simulink model "Dyn_6DoF_v2_0_R2015B"  (R2015b)
settings: Solver=ode4  SolverMode=SingleTasking  StartTime=0.0  StopTime=simInit.TSIM  FixedStep=simInit.dt  MaxStep=simInit.dt  RelTol=1e-3
InitFcn:
  | close all
undefined symbols (not defined in the file): act, base_windspeed, constr, DE2019, DiscIntNeverNeededParam, ENVMT, Lbooth, loiterStates, omega_rate_max, params, simInit, T, winchParameter
libraries: simulink x41, simulink_extras x4, dspsigops x1
(part 3 of 6)

== system Dyn_6DoF_v2_0_R2015B/AirborneSystem/FlightControlSystem/AttitudeAndRateLoop/AttitudeController/SecondOrderReferenceModel_alpha_a ==
  y_cmd : Inport
  hedge : Inport  Port=2
  Constant5 : Constant  Value=omega0_max
  Discrete-Time Integrator : DiscreteIntegrator  InitialConditionSetting=State (most efficient)  SampleTime=-1  LimitOutput=on  UpperSaturationLimit=y_max  LowerSaturationLimit=y_min  ICPrevOutput=DiscIntNeverNeededParam  ICPrevScaledInput=DiscIntNeverNeededParam
  Discrete-Time Integrator1 : DiscreteIntegrator  InitialConditionSetting=State (most efficient)  SampleTime=-1  LimitOutput=on  UpperSaturationLimit=yd_max  LowerSaturationLimit=yd_min  ICPrevOutput=DiscIntNeverNeededParam  ICPrevScaledInput=DiscIntNeverNeededParam
  Gain2 : Gain  Gain=2*zeta0
  Product : Product  Inputs=3
  Product1 : Product
  Saturation : Saturate  UpperLimit=y_max  LowerLimit=y_min
  Saturation1 : Saturate  UpperLimit=y2d_max  LowerLimit=y2d_min
  Sum : Sum  Inputs=|+-
  Sum1 : Sum  Inputs=|+-
  Sum2 : Sum  Inputs=|+-
  y_ref : Outport
  y_ref_dot : Outport  Port=2
  wires:
  Product/1 -> Sum/1
  Sum/1 -> Saturation1/1
  y_cmd/1 -> Saturation/1
  Saturation1/1 -> Discrete-Time Integrator1/1
  Gain2/1 -> Sum/2
  Sum1/1 -> Product/2
  Discrete-Time Integrator/1 -> Sum1/2, y_ref/1
  Discrete-Time Integrator1/1 -> y_ref_dot/1, Product1/1, Sum2/1
  Saturation/1 -> Sum1/1
  Sum2/1 -> Discrete-Time Integrator/1
  hedge/1 -> Sum2/2
  Product1/1 -> Gain2/1
  Constant5/1 -> Product1/2, Product/3, Product/1

== system Dyn_6DoF_v2_0_R2015B/AirborneSystem/FlightControlSystem/AttitudeAndRateLoop/AttitudeController/SecondOrderReferenceModel_mu_a ==
  y_cmd : Inport
  hedge : Inport  Port=2
  Constant5 : Constant  Value=omega0_max
  Discrete-Time Integrator : DiscreteIntegrator  InitialConditionSetting=State (most efficient)  SampleTime=-1  LimitOutput=on  UpperSaturationLimit=y_max  LowerSaturationLimit=y_min  ICPrevOutput=DiscIntNeverNeededParam  ICPrevScaledInput=DiscIntNeverNeededParam
  Discrete-Time Integrator1 : DiscreteIntegrator  InitialConditionSetting=State (most efficient)  SampleTime=-1  LimitOutput=on  UpperSaturationLimit=yd_max  LowerSaturationLimit=yd_min  ICPrevOutput=DiscIntNeverNeededParam  ICPrevScaledInput=DiscIntNeverNeededParam
  Gain2 : Gain  Gain=2*zeta0
  Product : Product  Inputs=3
  Product1 : Product
  Saturation : Saturate  UpperLimit=y_max  LowerLimit=y_min
  Saturation1 : Saturate  UpperLimit=y2d_max  LowerLimit=y2d_min
  Sum : Sum  Inputs=|+-
  Sum1 : Sum  Inputs=|+-
  Sum2 : Sum  Inputs=|+-
  y_ref : Outport
  y_ref_dot : Outport  Port=2
  wires:
  Discrete-Time Integrator/1 -> Sum1/2, y_ref/1
  Product/1 -> Sum/1
  y_cmd/1 -> Saturation/1
  Discrete-Time Integrator1/1 -> y_ref_dot/1, Product1/1, Sum2/1
  Sum/1 -> Saturation1/1
  Gain2/1 -> Sum/2
  Sum1/1 -> Product/2
  Saturation1/1 -> Discrete-Time Integrator1/1
  Saturation/1 -> Sum1/1
  Sum2/1 -> Discrete-Time Integrator/1
  hedge/1 -> Sum2/2
  Product1/1 -> Gain2/1
  Constant5/1 -> Product1/2, Product/3, Product/1

== system Dyn_6DoF_v2_0_R2015B/AirborneSystem/FlightControlSystem/AttitudeAndRateLoop/RateLoop/Actuatormodel _SS_2 ==
  u_cmd : Inport
  Aileron1 : Subsystem  mask(Rate and Position Limited Servo){freq=act.aileron.w0/(2*pi), RL=act.aileron.rl, POS_hi=act.aileron.max_deflection, POS_lo=act.aileron.min_deflection, Bias=act.aileron.bias}
      mask prompts: freq "Bandwidth, Hz"; RL "Rate Limit:"; POS_hi "Position Limit High:"; POS_lo "Position Limit Low:"; Bias "Bias Value:"
      mask help:
      | First order transfer function: w/(s+w), with rate and position limits
      | and output bias level.
      mask Display:
      | text(.48,.55,sprintf('%3.1f Hz\nBW',freq),'horizontalAlignment','center');
      | 
      | text(0.18,0.45,sprintf('|d/dt|\n<%0.1f',RL),'horizontalAlignment','center');
      | 
      | text(0.88,0.85,num2str(POS_hi),'horizontalAlignment', 'center');
      | text(0.88,0.2,num2str(POS_lo),'horizontalAlignment', 'center');
      | text(0.73,0.5,'P\nL');
      | 
      | 
      | plot([0.83 0.87 0.93 0.97],[0.4 0.4 0.6 0.6]);
      | plot([0.81 0.99],[0.5 0.5]);
      | plot([0.9 0.9],[0.3 0.7]);
      | plot([0.81 0.99 0.99 0.81 0.81],[0.3 0.3 0.7 0.7 0.3]);
  Delay1 : Delay  Commented=on  DelayLength=1  InitialCondition=0
  Delay2 : Delay  Commented=on  DelayLength=1  InitialCondition=0
  Delay3 : Delay  Commented=on  DelayLength=1  InitialCondition=0
  Delay4 : Delay  DelayLength=1  InitialCondition=0
  Delay5 : Delay  DelayLength=1  InitialCondition=0
  Delay6 : Delay  DelayLength=1  InitialCondition=0
  Demux : Demux  Outputs=3
  Elevator : Subsystem  mask(Rate and Position Limited Servo){freq=act.elevator.w0/(2*pi), RL=act.elevator.rl, POS_hi=act.elevator.max_deflection, POS_lo=act.elevator.min_deflection, Bias=act.elevator.bias}
      mask prompts: freq "Bandwidth, Hz"; RL "Rate Limit:"; POS_hi "Position Limit High:"; POS_lo "Position Limit Low:"; Bias "Bias Value:"
      mask help:
      | First order transfer function: w/(s+w), with rate and position limits
      | and output bias level.
      mask Display:
      | text(.48,.55,sprintf('%3.1f Hz\nBW',freq),'horizontalAlignment','center');
      | 
      | text(0.18,0.45,sprintf('|d/dt|\n<%0.1f',RL),'horizontalAlignment','center');
      | 
      | text(0.88,0.85,num2str(POS_hi),'horizontalAlignment', 'center');
      | text(0.88,0.2,num2str(POS_lo),'horizontalAlignment', 'center');
      | text(0.73,0.5,'P\nL');
      | 
      | 
      | plot([0.83 0.87 0.93 0.97],[0.4 0.4 0.6 0.6]);
      | plot([0.81 0.99],[0.5 0.5]);
      | plot([0.9 0.9],[0.3 0.7]);
      | plot([0.81 0.99 0.99 0.81 0.81],[0.3 0.3 0.7 0.7 0.3]);
  Manual Switch : ManualSwitch  CurrentSetting=0
  Mux1 : Mux  Inputs=3
  Mux2 : Mux  Inputs=3
  Rudder1 : Subsystem  mask(Rate and Position Limited Servo){freq=act.rudder.w0/(2*pi), RL=act.rudder.rl, POS_hi=act.rudder.max_deflection, POS_lo=act.rudder.min_deflection, Bias=act.rudder.bias}
      mask prompts: freq "Bandwidth, Hz"; RL "Rate Limit:"; POS_hi "Position Limit High:"; POS_lo "Position Limit Low:"; Bias "Bias Value:"
      mask help:
      | First order transfer function: w/(s+w), with rate and position limits
      | and output bias level.
      mask Display:
      | text(.48,.55,sprintf('%3.1f Hz\nBW',freq),'horizontalAlignment','center');
      | 
      | text(0.18,0.45,sprintf('|d/dt|\n<%0.1f',RL),'horizontalAlignment','center');
      | 
      | text(0.88,0.85,num2str(POS_hi),'horizontalAlignment', 'center');
      | text(0.88,0.2,num2str(POS_lo),'horizontalAlignment', 'center');
      | text(0.73,0.5,'P\nL');
      | 
      | 
      | plot([0.83 0.87 0.93 0.97],[0.4 0.4 0.6 0.6]);
      | plot([0.81 0.99],[0.5 0.5]);
      | plot([0.9 0.9],[0.3 0.7]);
      | plot([0.81 0.99 0.99 0.81 0.81],[0.3 0.3 0.7 0.7 0.3]);
  Saturation : Saturate  Commented=on  UpperLimit=act.aileron.max_deflection  LowerLimit=act.aileron.min_deflection
  Saturation1 : Saturate  Commented=on  UpperLimit=act.elevator.max_deflection  LowerLimit=act.elevator.min_deflection
  Saturation2 : Saturate  Commented=on  UpperLimit=act.rudder.max_deflection  LowerLimit=act.rudder.min_deflection
  Saturation4 : Saturate  UpperLimit=act.elevator.max_deflection  LowerLimit=act.elevator.min_deflection
  Saturation6 : Saturate  UpperLimit=act.aileron.max_deflection  LowerLimit=act.aileron.min_deflection
  Saturation7 : Saturate  UpperLimit=act.rudder.max_deflection  LowerLimit=act.rudder.min_deflection
  Act_out_est : Outport
  wires:
  Delay3/1 -> Saturation2/1
  Mux2/1 -> Manual Switch/2
  Saturation1/1 -> Mux1/2
  Delay4/1 -> Saturation6/1
  Delay1/1 -> Saturation/1
  Manual Switch/1 -> Act_out_est/1
  Saturation6/1 -> Aileron1/1(In)
  Saturation/1 -> Mux1/1
  Saturation7/1 -> Rudder1/1(In)
  Rudder1/1(Out) -> Mux2/3
  Elevator/1(Out) -> Mux2/2
  Delay5/1 -> Saturation4/1
  Demux/2 -> Delay5/1, Delay2/1
  Mux1/1 -> Manual Switch/1
  Demux/1 -> Delay1/1, Delay4/1
  Delay6/1 -> Saturation7/1
  Delay2/1 -> Saturation1/1
  Saturation4/1 -> Elevator/1(In)
  Saturation2/1 -> Mux1/3
  u_cmd/1 -> Demux/1
  Aileron1/1(Out) -> Mux2/1
  Demux/3 -> Delay6/1, Delay3/1

== system Dyn_6DoF_v2_0_R2015B/AirborneSystem/FlightControlSystem/AttitudeAndRateLoop/RateLoop/ControlAllocation ==
  deflections_actuator_output : Inport
  airdata : Inport  Port=2
  Delta_mom_cmd : Inport  Port=3
  Constant1 : Constant  Value=1e-6
  Gain14 : Gain  Gain=[1/ DE2019.b, 0, 0; 0, 1/ DE2019.c, 0; 0, 0, 1/ DE2019.b]  Multiplication=Matrix(K*u)
  Gain15 : Gain  Gain=DE2019.S_wing
  Gain3 : Gain  Gain=0.5*ENVMT.rhos
  Product : Product  Inputs=*/
  Product2 : Product
  Selector : Selector  InputPortWidth=3  IndexOptions=Index vector (dialog)  Indices=1  OutputSizes=1
  Selector1 : Selector  InputPortWidth=3  IndexOptions=Index vector (dialog)  Indices=2  OutputSizes=1
  Sum13 : Sum
  Sum2 : Sum  Inputs=|++
  allocation : MATLAB Function  TreatAsAtomicUnit=on
  deflections_cmd : Outport
  wires:
  Selector1/1 -> allocation/2(alpha)
  airdata/1 -> Selector/1, Selector1/1
  Product2/1 -> Gain3/1
  Selector/1 -> Product2/1, Product2/2
  deflections_actuator_output/1 -> Sum13/1
  Gain14/1 -> allocation/1(dC_pqr)
  Sum13/1 -> deflections_cmd/1
  allocation/1(Delta_deltas) -> Sum13/2
  Sum2/1 -> Product/2
  Constant1/1 -> Sum2/2
  Gain3/1 -> Gain15/1
  Gain15/1 -> Sum2/1
  Product/1 -> Gain14/1
  Delta_mom_cmd/1 -> Product/1

== system Dyn_6DoF_v2_0_R2015B/AirborneSystem/FlightControlSystem/AttitudeAndRateLoop/RateLoop/Rate_Loop ==
  omega_OB_B : Inport
  omega_OB_B_cmd : Inport  Port=2  PortDimensions=[3,1]
  M_a_B_est : Inport  Port=3  PortDimensions=[3,1]
  Demux1 : Demux  Commented=on  Outputs=3
  Demux2 : Demux  Commented=on  Outputs=3
  Demux3 : Demux  Commented=on  Outputs=3
  Gain : Gain  Commented=on  Gain=180/pi
  Gain1 : Gain  Commented=on  Gain=180/pi
  Gain2 : Gain  Commented=on  Gain=180/pi
  Hedging : Subsystem
  InversionRotationalDynamics : MATLAB Function  TreatAsAtomicUnit=on
  Mux{,1..2,4} (4 alike) : Mux  Commented=on  Inputs=3
  NonlinearDynamicInversion : Subsystem
  Scope : Scope  Commented=on  NumInputPorts=3
  Selector : Selector  InputPortWidth=3  IndexOptions=Index vector (dialog)  Indices=1  OutputSizes=1
  Selector1 : Selector  InputPortWidth=3  IndexOptions=Index vector (dialog)  Indices=2  OutputSizes=1
  Selector2 : Selector  InputPortWidth=3  IndexOptions=Index vector (dialog)  Indices=3  OutputSizes=1
  Sum1 : Sum  Inputs=|+-
  Sum12 : Sum  Inputs=-+
  Sum2 : Sum  Inputs=|+-
  Sum3 : Sum  Inputs=|+-
  To Workspace11 : ToWorkspace  Commented=on  VariableName=omega_OB_B_cmds  SaveFormat=Timeseries  SampleTime=-1
  delta_M_cmd : Outport
  wires:
  Mux2/1 -> To Workspace11/1
  omega_OB_B_cmd/1 -> Demux2/1, NonlinearDynamicInversion/5(omega_OB_B_cmd)
  Selector/1 -> Sum2/1
  Selector1/1 -> Sum1/1
  Selector2/1 -> Sum3/1
  NonlinearDynamicInversion/1(omega_OB_ref) -> Demux1/1
  Sum3/1 -> NonlinearDynamicInversion/1(r_h)
  Sum1/1 -> NonlinearDynamicInversion/2(q_h)
  Sum2/1 -> NonlinearDynamicInversion/3(p_h)
  Hedging/3(nu_r_hat) -> Sum3/2
  Hedging/2(nu_q_hat) -> Sum1/2
  Hedging/1(nu_p_hat) -> Sum2/2
  Sum12/1 -> delta_M_cmd/1
  InversionRotationalDynamics/1(M_des) -> Sum12/2
  M_a_B_est/1 -> Hedging/1(Torque_estimate), Sum12/1
  Gain1/1 -> Scope/2
  Mux/1 -> Gain/1, Mux2/1
  Mux1/1 -> Gain1/1, Mux2/2
  Demux1/1 -> Mux/2
  Demux1/2 -> Mux1/2
  Demux1/3 -> Mux4/2
  Mux4/1 -> Gain2/1, Mux2/3
  Gain2/1 -> Scope/3
  Gain/1 -> Scope/1
  Demux2/1 -> Mux/1
  Demux2/2 -> Mux1/1
  Demux2/3 -> Mux4/1
  Demux3/1 -> Mux/3
  Demux3/2 -> Mux1/3
  Demux3/3 -> Mux4/3
  omega_OB_B/1 -> Demux3/1, Hedging/2(rates), InversionRotationalDynamics/1(omega_OB_B), NonlinearDynamicInversion/4(omega_OB_B)
  NonlinearDynamicInversion/2(nu_NDI) -> Selector/1, Selector1/1, Selector2/1, InversionRotationalDynamics/2(nu_NDI)

== system Dyn_6DoF_v2_0_R2015B/AirborneSystem/FlightControlSystem/PathFollowingController_SS_3/FlightOnFlatEarth (Retraction&Loitering)/CalculateAttitudeCmds ==
  flight_on_flatearth_flag : Inport
  pathangles_k_cmd : Inport  Port=2
  Ft_set : Inport  Port=3
  F_t_kite : Inport  Port=4
  sub_flightMode : Inport  Port=5
  flightMode : Inport  Port=6
  StateEstimation_Bus : Inport  Port=7
  Demux : Demux  Outputs=3
  FlightPathLoopRetraction_Aerodynamic : Subsystem
  Mux1 : Mux  Inputs=3
  Signal Specification : SignalSpecification  Dimensions=[3,1]
  Terminator2 : Terminator
  mu_a_cmd : Outport
  alpha_cmd : Outport  Port=2
  wires:
  StateEstimation_Bus/1 -> FlightPathLoopRetraction_Aerodynamic/4(StateEstimation_Bus)
  Demux/3 -> Terminator2/1
  Demux/2 -> alpha_cmd/1
  flight_on_flatearth_flag/1 -> FlightPathLoopRetraction_Aerodynamic/Enable
  FlightPathLoopRetraction_Aerodynamic/2(alpha_a_cmd) -> Mux1/2
  flightMode/1 -> FlightPathLoopRetraction_Aerodynamic/1(flight_mode)
  Signal Specification/1 -> Demux/1
  Demux/1 -> mu_a_cmd/1
  Mux1/1 -> Signal Specification/1
  F_t_kite/1 -> FlightPathLoopRetraction_Aerodynamic/3(F_t_kite)
  FlightPathLoopRetraction_Aerodynamic/1(mu_a_cmd) -> Mux1/1
  Ft_set/1 -> FlightPathLoopRetraction_Aerodynamic/2(F_t_set)
  FlightPathLoopRetraction_Aerodynamic/3(beta_a_cmd) -> Mux1/3
  pathangles_k_cmd/1 -> FlightPathLoopRetraction_Aerodynamic/5(kinematic_path_cmd)
  sub_flightMode/1 -> FlightPathLoopRetraction_Aerodynamic/6(sub_flightMode)

== system Dyn_6DoF_v2_0_R2015B/AirborneSystem/FlightControlSystem/PathFollowingController_SS_3/FlightOnFlatEarth (Retraction&Loitering)/GuidanceFlatEarth ==
  flightMode : Inport
  StateEstimation_Bus : Inport  Port=2
  reset_flat : Inport  Port=3
  V_ro : Inport  Port=4
  Tether_length : Inport  Port=5
  Enable : EnablePort
  Bus Selector : BusSelector  OutputSignals=pos_G_O_m,vel_K_O_mDs,pathangles_k,pos_G_W
  Compare To Constant : simulink/Logic and Bit Operations/Compare To Constant  relop===  const=6  OutDataTypeStr=boolean
  Compare To Constant2 : simulink/Logic and Bit Operations/Compare To Constant  relop===  const=6  OutDataTypeStr=boolean
  LoiteringGuidance : Subsystem
  Retraction_Nav : Subsystem
  Switch1 : Switch  Criteria=u2 > Threshold
  distances2slope : Outport
  course_path : Outport  Port=2
  valid_transition_region : Outport  Port=3
  transition_flag : Outport  Port=4
  flag_pos_W : Outport  Port=5
  transition_x_target : Outport  Port=6
  Vk_desired_retraction : Outport  Port=7
  arcP : Outport  Port=8
  wires:
  Bus Selector/1 -> Retraction_Nav/1(pos_O), LoiteringGuidance/2(pos_G_O_m)  "<pos_G_O_m>"
  StateEstimation_Bus/1 -> Bus Selector/1
  Bus Selector/2 -> Retraction_Nav/2(vel_k_O), LoiteringGuidance/3(vel_K_O_mDs)  "<vel_K_O_mDs>"
  Compare To Constant2/1 -> Retraction_Nav/Enable
  Switch1/1 -> course_path/1
  Compare To Constant/1 -> Switch1/2
  Retraction_Nav/1(distances2slope) -> distances2slope/1
  Retraction_Nav/7(path_k_cmds) -> Switch1/1
  flightMode/1 -> LoiteringGuidance/1(flightMode), Compare To Constant/1, Compare To Constant2/1
  Bus Selector/3 -> LoiteringGuidance/4(pathangles_k)  "<pathangles_k>"
  LoiteringGuidance/1(path_k_cmds) -> Switch1/3
  LoiteringGuidance/2(valid_transition_region) -> valid_transition_region/1
  Retraction_Nav/2(transition_flag) -> transition_flag/1
  reset_flat/1 -> LoiteringGuidance/6(reset_flag)
  Bus Selector/4 -> LoiteringGuidance/5(pos_W)  "<pos_G_W>"
  Retraction_Nav/3(flag_pos_y_W) -> flag_pos_W/1
  Retraction_Nav/4(transition_x_target) -> transition_x_target/1
  Retraction_Nav/5(Vk_desired_retraction) -> Vk_desired_retraction/1
  V_ro/1 -> Retraction_Nav/3(V_ro)
  Tether_length/1 -> Retraction_Nav/4(Tether_length)
  Retraction_Nav/6(arcP) -> arcP/1

== system Dyn_6DoF_v2_0_R2015B/AirborneSystem/FlightControlSystem/PathFollowingController_SS_3/FlightOnSphere (Traction)/FlightPathLoopTraction ==
  Ft_set : Inport
  F_a_B_est : Inport  Port=2  PortDimensions=[3,1]
  StateEstimation_Bus : Inport  Port=3
  nu_chi : Inport  Port=4
  nu_gamma : Inport  Port=5
  Enable : EnablePort  StatesWhenEnabling=reset
  Bus Selector : BusSelector  OutputSignals=pos_G_O_m,pathangles_k,v_k_B,airdata,mu_a
  Delay : Delay  DelayLength=1  InitialConditionSource=Input port
      settings: InputPortMap=u0,p4
  Delay1 : Delay  DelayLength=1  InitialConditionSource=Input port
      settings: InputPortMap=u0,p4
  Delay{2..5} (4 alike) : Delay  DelayLength=1
  Demux : Demux  Outputs=2
  Demux1 : Demux  Outputs=2
  Demux2 : Demux  Outputs=2
  EstimatePlantResponse : Subsystem
  MATLAB Function : MATLAB Function  TreatAsAtomicUnit=on
  Mux : Mux  Inputs=2
  Saturation : Saturate  UpperLimit=constr.alpha_a_max  LowerLimit=constr.alpha_a_min
  Sum{,1..3} (4 alike) : Sum  Inputs=|+-
  inversionPathDynamics : MATLAB Function  TreatAsAtomicUnit=on
  mu_a_c_traction : Outport  PortDimensions=1
  alpha_rq : Outport  Port=2  PortDimensions=1
  wires:
  Bus Selector/5 -> Delay/2  "<mu_a>"
  F_a_B_est/1 -> inversionPathDynamics/4(F_a_B_est)
  Demux1/1 -> inversionPathDynamics/6(chi_k)
  inversionPathDynamics/1(mu_a) -> Delay/1, mu_a_c_traction/1
  Mux/1 -> Demux/1
  Demux/2 -> inversionPathDynamics/3(nu_gamma_k)
  Demux/1 -> inversionPathDynamics/2(nu_chi_k)
  inversionPathDynamics/2(mu_k_c) -> EstimatePlantResponse/3(mu_k_sat)
  inversionPathDynamics/3(alpha_rq) -> Saturation/1
  Saturation/1 -> alpha_rq/1, EstimatePlantResponse/2(alpha_rq)
  inversionPathDynamics/4(dphi) -> EstimatePlantResponse/1(dphi)
  Delay1/1 -> inversionPathDynamics/10(L_rq_old)
  Delay/1 -> inversionPathDynamics/11(mu_a_old)
  MATLAB Function/1(L_rq) -> Delay1/2
  inversionPathDynamics/5(L_rq) -> Delay1/1
  Demux1/2 -> inversionPathDynamics/7(gamma_k)
  StateEstimation_Bus/1 -> EstimatePlantResponse/5(StateEstimation_Bus), Bus Selector/1
  Bus Selector/4 -> inversionPathDynamics/9(airdata), MATLAB Function/1(airdata)  "<airdata>"
  Bus Selector/2 -> Demux1/1  "<pathangles_k>"
  Bus Selector/3 -> inversionPathDynamics/8(v_k_B)  "<v_k_B>"
  Bus Selector/1 -> inversionPathDynamics/5(pos_O)  "<pos_G_O_m>"
  Delay5/1 -> Sum3/1
  nu_chi/1 -> Sum/1
  Sum3/1 -> Sum/2
  Delay4/1 -> Sum2/2
  Delay3/1 -> Sum3/2
  Demux2/2 -> Delay4/1
  Sum1/1 -> Mux/2, Delay2/1
  Sum/1 -> Mux/1, Delay5/1
  Delay2/1 -> Sum2/1
  EstimatePlantResponse/1(pathAngleRate) -> Demux2/1
  nu_gamma/1 -> Sum1/1
  Demux2/1 -> Delay3/1
  Sum2/1 -> Sum1/2
  Ft_set/1 -> EstimatePlantResponse/4(Ft), inversionPathDynamics/1(Ft_set)

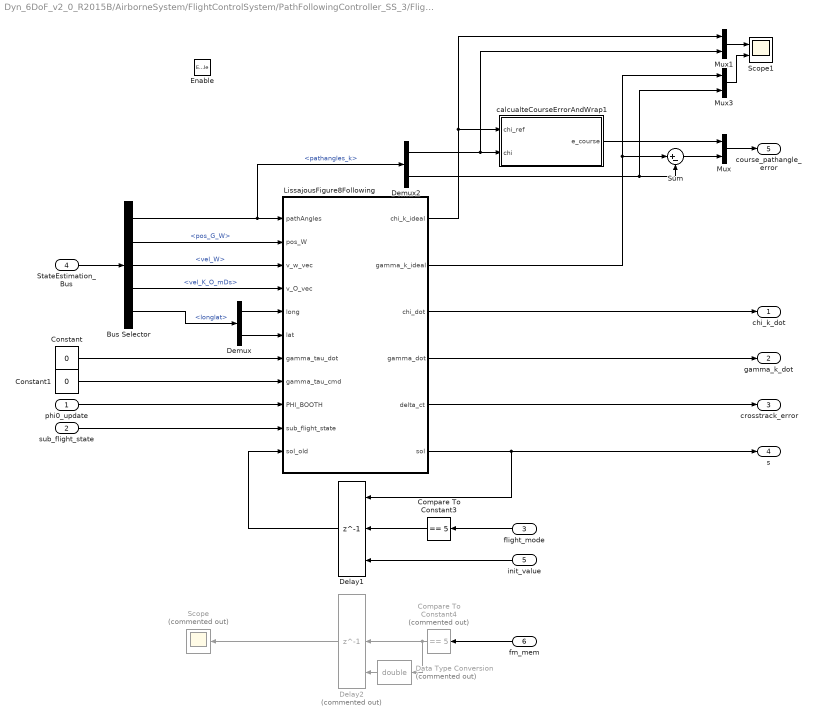
== system Dyn_6DoF_v2_0_R2015B/AirborneSystem/FlightControlSystem/PathFollowingController_SS_3/FlightOnSphere (Traction)/Navigator ==
  phi0_update : Inport
  sub_flight_state : Inport  Port=2
  flight_mode : Inport  Port=3
  StateEstimation_Bus : Inport  Port=4
  init_value : Inport  Port=5
  fm_mem : Inport  Port=6
  Enable : EnablePort  StatesWhenEnabling=reset
  Bus Selector : BusSelector  OutputSignals=pathangles_k,pos_G_W,vel_W,vel_K_O_mDs,longlat
  Compare To Constant3 : simulink/Logic and Bit Operations/Compare To Constant  relop===  const=5  OutDataTypeStr=boolean
  Compare To Constant4 : simulink/Logic and Bit Operations/Compare To Constant  Commented=on  relop===  const=5  OutDataTypeStr=boolean
  Constant : Constant  Value=0
  Constant1 : Constant  Value=0
  Data Type Conversion : DataTypeConversion  Commented=on  OutDataTypeStr=double
  Delay1 : Delay  DelayLength=1  InitialConditionSource=Input port  InitialCondition=pi/2  ExternalReset=Rising
      settings: InputPortMap=u0,r5,p4
  Delay2 : Delay  Commented=on  DelayLength=1  InitialConditionSource=Input port  InitialCondition=pi/2  ExternalReset=Rising
      settings: InputPortMap=u0,r5,p4
  Demux : Demux  Outputs=2
  Demux2 : Demux  Outputs=2
  LissajousFigure8Following : MATLAB Function  TreatAsAtomicUnit=on
  Mux : Mux  Inputs=2
  Mux1 : Mux  Inputs=2
  Mux3 : Mux  Inputs=2
  Scope : Scope  Commented=on
  Scope1 : Scope  NumInputPorts=2
  Sum : Sum  Inputs=|+-
  calcualteCourseErrorAndWrap1 : MATLAB Function  TreatAsAtomicUnit=on
  chi_k_dot : Outport  PortDimensions=1
  gamma_k_dot : Outport  Port=2  PortDimensions=1
  crosstrack_error : Outport  Port=3
  s : Outport  Port=4  PortDimensions=1  InitialOutput=0
  course_pathangle_error : Outport  Port=5
  wires:
  Mux3/1 -> Scope1/2
  Mux1/1 -> Scope1/1
  Delay1/1 -> LissajousFigure8Following/11(sol_old)
  LissajousFigure8Following/6(sol) -> s/1, Delay1/1
  Bus Selector/4 -> LissajousFigure8Following/4(v_O_vec)  "<vel_K_O_mDs>"
  Demux/1 -> LissajousFigure8Following/5(long)
  calcualteCourseErrorAndWrap1/1(e_course) -> Mux/1
  LissajousFigure8Following/1(chi_k_ideal) -> calcualteCourseErrorAndWrap1/1(chi_ref), Mux1/1
  LissajousFigure8Following/2(gamma_k_ideal) -> Sum/1, Mux3/1
  Demux2/1 -> Mux1/2, calcualteCourseErrorAndWrap1/2(chi)
  Demux2/2 -> Mux3/2, Sum/2
  Mux/1 -> course_pathangle_error/1
  LissajousFigure8Following/4(gamma_dot) -> gamma_k_dot/1
  LissajousFigure8Following/3(chi_dot) -> chi_k_dot/1
  Sum/1 -> Mux/2
  Demux/2 -> LissajousFigure8Following/6(lat)
  LissajousFigure8Following/5(delta_ct) -> crosstrack_error/1
  StateEstimation_Bus/1 -> Bus Selector/1
  Bus Selector/2 -> LissajousFigure8Following/2(pos_W)  "<pos_G_W>"
  Bus Selector/5 -> Demux/1  "<longlat>"
  Bus Selector/1 -> Demux2/1, LissajousFigure8Following/1(pathAngles)  "<pathangles_k>"
  flight_mode/1 -> Compare To Constant3/1
  phi0_update/1 -> LissajousFigure8Following/9(PHI_BOOTH)
  Compare To Constant3/1 -> Delay1/2
  init_value/1 -> Delay1/3
  Constant/1 -> LissajousFigure8Following/7(gamma_tau_dot)
  Bus Selector/3 -> LissajousFigure8Following/3(v_w_vec)  "<vel_W>"
  Constant1/1 -> LissajousFigure8Following/8(gamma_tau_cmd)
  Delay2/1 -> Scope/1
  Compare To Constant4/1 -> Delay2/2, Data Type Conversion/1
  fm_mem/1 -> Compare To Constant4/1
  Data Type Conversion/1 -> Delay2/3
  sub_flight_state/1 -> LissajousFigure8Following/10(sub_flight_state)

== system Dyn_6DoF_v2_0_R2015B/AirborneSystem/FlightControlSystem/PathFollowingController_SS_3/FlightOnSphere (Traction)/Pcontroller_ChiGamma_Traction ==
  course_pathangle_error : Inport
  Demux : Demux  Outputs=2
  Kp : Gain  Gain=params.Kp_gamma_k_traction  Multiplication=Matrix(K*u)
  Kp1 : Gain  Gain=params.Kp_chi_k_traction  Multiplication=Matrix(K*u)
  Chi_cntr : Outport
  Gamma_cntr : Outport  Port=2
  wires:
  Kp1/1 -> Chi_cntr/1
  Kp/1 -> Gamma_cntr/1
  course_pathangle_error/1 -> Demux/1
  Demux/2 -> Kp/1
  Demux/1 -> Kp1/1

== system Dyn_6DoF_v2_0_R2015B/AirborneSystem/ForcesAndTorques/aerodynamic forces FSI/Wing Aero/If Action Subsystem ==
  FSI_in : Inport
  simTime : Inport  Port=2
  Action Port : ActionPort
  Demux1 : Demux  Outputs=6
  FSI_sim : MATLABFcn  Commented=on  MATLABFcn=Init_FSIsim  OutputDimensions=[6,1]  Output1D=off
  MATLAB Function : MATLAB Function  TreatAsAtomicUnit=on
  Mux6 : Mux  Inputs=2
  Terminator{1..5,7} (6 alike) : Terminator  Commented=on
  FSI_out : Outport
  wires:
  Demux1/1 -> Terminator7/1  "Fx"
  Demux1/6 -> Terminator1/1  "Myaw"
  simTime/1 -> Mux6/2
  Mux6/1 -> MATLAB Function/1(u)
  Demux1/5 -> Terminator2/1  "Mpitch"
  Demux1/2 -> Terminator3/1  "Fy"
  FSI_in/1 -> Mux6/1
  MATLAB Function/1(y) -> FSI_out/1, Demux1/1
  Demux1/3 -> Terminator5/1  "Fz"
  Demux1/4 -> Terminator4/1  "Mroll"

== system Dyn_6DoF_v2_0_R2015B/AirborneSystem/ForcesAndTorques/aerodynamic forces FSI/Wing Aero/If Action Subsystem1 ==
  Simple_in : Inport
  Action Port : ActionPort
  FSI : Subsystem
  Simple_out : Outport
  wires:
  Simple_in/1 -> FSI/1(In1)
  FSI/1(Out1) -> Simple_out/1

== system Dyn_6DoF_v2_0_R2015B/Environment_SS_5/Windshear/Wind Shear Model/wind_field_calc/Length Conversion ==
  in : Inport
  Unit Conversion : UnitConversion
  out : Outport
  wires:
  Unit Conversion/1 -> out/1
  in/1 -> Unit Conversion/1

== system Dyn_6DoF_v2_0_R2015B/AirborneSystem/FlightControlSystem/AttitudeAndRateLoop/RateLoop/Actuatormodel _SS_2/Aileron1 ==
  In : Inport
  Constant : Constant  Value=Bias
  Constant2 : Constant
  Discrete-Time Integrator : DiscreteIntegrator  InitialConditionSource=external  InitialConditionSetting=State (most efficient)  SampleTime=-1  LimitOutput=on  UpperSaturationLimit=POS_hi  LowerSaturationLimit=POS_lo  ICPrevOutput=DiscIntNeverNeededParam  ICPrevScaledInput=DiscIntNeverNeededParam
  Gain : Gain  Gain=2*pi*freq  SaturateOnIntegerOverflow=on  OutDataTypeStr=Inherit: Same as input  ParamDataTypeStr=Inherit: Same as input
  Product : Product
  Rate Limiter : Saturate  UpperLimit=RL  LowerLimit=-RL
  Sum : Sum  Inputs=-+|  SaturateOnIntegerOverflow=on  InputSameDT=on  OutDataTypeStr=Inherit: Same as first input
  Sum1 : Sum  Inputs=++|  SaturateOnIntegerOverflow=on  InputSameDT=on  OutDataTypeStr=Inherit: Same as first input
  Out : Outport  PortDimensions=1
  wires:
  Constant2/1 -> Product/1
  Constant/1 -> Sum1/1
  Gain/1 -> Product/2  "Ydot"
  Sum/1 -> Gain/1  "Error"
  Discrete-Time Integrator/1 -> Sum/1, Out/1  "Y"
  Rate Limiter/1 -> Discrete-Time Integrator/1  "Ydot_lim"
  In/1 -> Sum1/2
  Sum1/1 -> Sum/2, Discrete-Time Integrator/2
  Product/1 -> Rate Limiter/1

== system Dyn_6DoF_v2_0_R2015B/AirborneSystem/FlightControlSystem/AttitudeAndRateLoop/RateLoop/Actuatormodel _SS_2/Elevator ==
  In : Inport
  Constant : Constant  Value=Bias
  Discrete-Time Integrator : DiscreteIntegrator  InitialConditionSource=external  InitialConditionSetting=State (most efficient)  SampleTime=-1  LimitOutput=on  UpperSaturationLimit=POS_hi  LowerSaturationLimit=POS_lo  ICPrevOutput=DiscIntNeverNeededParam  ICPrevScaledInput=DiscIntNeverNeededParam
  Gain : Gain  Gain=2*pi*freq  SaturateOnIntegerOverflow=on  OutDataTypeStr=Inherit: Same as input  ParamDataTypeStr=Inherit: Same as input
  Rate Limiter : Saturate  UpperLimit=RL  LowerLimit=-RL
  Scope : Scope  NumInputPorts=2
  Sum : Sum  Inputs=-+|  SaturateOnIntegerOverflow=on  InputSameDT=on  OutDataTypeStr=Inherit: Same as first input
  Sum1 : Sum  Inputs=++|  SaturateOnIntegerOverflow=on  InputSameDT=on  OutDataTypeStr=Inherit: Same as first input
  Out : Outport  PortDimensions=1
  wires:
  Sum1/1 -> Discrete-Time Integrator/2, Sum/2
  In/1 -> Sum1/2
  Rate Limiter/1 -> Scope/2, Discrete-Time Integrator/1  "Ydot_lim"
  Discrete-Time Integrator/1 -> Out/1, Sum/1  "Y"
  Sum/1 -> Gain/1  "Error"
  Gain/1 -> Scope/1, Rate Limiter/1  "Ydot"
  Constant/1 -> Sum1/1

== system Dyn_6DoF_v2_0_R2015B/AirborneSystem/FlightControlSystem/AttitudeAndRateLoop/RateLoop/Actuatormodel _SS_2/Rudder1 ==
  In : Inport
  Constant : Constant  Value=Bias
  Discrete-Time Integrator : DiscreteIntegrator  InitialConditionSource=external  InitialConditionSetting=State (most efficient)  SampleTime=-1  LimitOutput=on  UpperSaturationLimit=POS_hi  LowerSaturationLimit=POS_lo  ICPrevOutput=DiscIntNeverNeededParam  ICPrevScaledInput=DiscIntNeverNeededParam
  Gain : Gain  Gain=2*pi*freq  SaturateOnIntegerOverflow=on  OutDataTypeStr=Inherit: Same as input  ParamDataTypeStr=Inherit: Same as input
  Rate Limiter : Saturate  UpperLimit=RL  LowerLimit=-RL
  Sum : Sum  Inputs=-+|  SaturateOnIntegerOverflow=on  InputSameDT=on  OutDataTypeStr=Inherit: Same as first input
  Sum1 : Sum  Inputs=++|  SaturateOnIntegerOverflow=on  InputSameDT=on  OutDataTypeStr=Inherit: Same as first input
  Out : Outport  PortDimensions=1
  wires:
  Constant/1 -> Sum1/1
  Sum1/1 -> Discrete-Time Integrator/2, Sum/2
  In/1 -> Sum1/2
  Rate Limiter/1 -> Discrete-Time Integrator/1  "Ydot_lim"
  Discrete-Time Integrator/1 -> Out/1, Sum/1  "Y"
  Sum/1 -> Gain/1  "Error"
  Gain/1 -> Rate Limiter/1  "Ydot"

== system Dyn_6DoF_v2_0_R2015B/AirborneSystem/FlightControlSystem/AttitudeAndRateLoop/RateLoop/Rate_Loop/Hedging ==
  Torque_estimate : Inport
  rates : Inport  Port=2
  Demux1 : Demux  Outputs=3
  InversionRotationalDynamics1 : MATLAB Function  TreatAsAtomicUnit=on
  Signal Specification : SignalSpecification  Dimensions=[3,1]
  nu_p_hat : Outport
  nu_q_hat : Outport  Port=2
  nu_r_hat : Outport  Port=3
  wires:
  Signal Specification/1 -> InversionRotationalDynamics1/1(Moments)
  Torque_estimate/1 -> Signal Specification/1
  InversionRotationalDynamics1/3(nu_r_hat) -> nu_r_hat/1
  InversionRotationalDynamics1/2(nu_q_hat) -> nu_q_hat/1
  rates/1 -> Demux1/1
  InversionRotationalDynamics1/1(nu_p_hat) -> nu_p_hat/1
  Demux1/2 -> InversionRotationalDynamics1/3(q)
  Demux1/1 -> InversionRotationalDynamics1/2(p)
  Demux1/3 -> InversionRotationalDynamics1/4(r)

== system Dyn_6DoF_v2_0_R2015B/AirborneSystem/FlightControlSystem/AttitudeAndRateLoop/RateLoop/Rate_Loop/NonlinearDynamicInversion ==
  r_h : Inport
  q_h : Inport  Port=2
  p_h : Inport  Port=3
  omega_OB_B : Inport  Port=4
  omega_OB_B_cmd : Inport  Port=5
  Demux3 : Demux  Outputs=3
  Mux : Mux  Inputs=3
  Mux1 : Mux  Commented=on  Inputs=2
  Mux2 : Mux  Inputs=3
  Mux3 : Mux  Commented=on  Inputs=2
  Mux4 : Mux  Commented=on  Inputs=2
  Scope3 : Scope  Commented=on  NumInputPorts=3
  Selector : Selector  InputPortWidth=3  IndexOptions=Index vector (dialog)  Indices=1  OutputSizes=1
  Selector1 : Selector  InputPortWidth=3  IndexOptions=Index vector (dialog)  Indices=2  OutputSizes=1
  Selector2 : Selector  InputPortWidth=3  IndexOptions=Index vector (dialog)  Indices=3  OutputSizes=1
  Subsystem2 : Subsystem  mask{w0_max=params.w0_p_max, Kp=params.Kp_p, Ki=0}
      mask prompts: w0_max "omega0_max"
  Subsystem7 : Subsystem  mask{w0_max=params.w0_q_max, Kp=params.Kp_q, Ki=0}
      mask prompts: w0_max "omega0_max"
  Subsystem8 : Subsystem  mask{w0_max=params.w0_r_max, Kp=params.Kp_r, Ki=0}
      mask prompts: w0_max "omega0_max"
  omega_OB_ref : Outport
  nu_NDI : Outport  Port=2
  wires:
  omega_OB_B_cmd/1 -> Demux3/1
  Mux/1 -> omega_OB_ref/1
  Demux3/1 -> Subsystem2/1(y_cmd), Mux1/1
  omega_OB_B/1 -> Selector2/1, Selector1/1, Selector/1
  Demux3/2 -> Subsystem7/1(y_cmd), Mux3/1
  Demux3/3 -> Subsystem8/1(y_cmd), Mux4/1
  Mux2/1 -> nu_NDI/1
  Mux1/1 -> Scope3/1
  Mux3/1 -> Scope3/2
  Mux4/1 -> Scope3/3
  Subsystem2/1(y_ref) -> Mux1/2, Mux/1
  p_h/1 -> Subsystem2/2(hedge)
  Subsystem2/2(nu_e) -> Mux2/1
  Subsystem7/1(y_ref) -> Mux3/2, Mux/2
  q_h/1 -> Subsystem7/2(hedge)
  Subsystem7/2(nu_e) -> Mux2/2
  Subsystem8/1(y_ref) -> Mux4/2, Mux/3
  r_h/1 -> Subsystem8/2(hedge)
  Subsystem8/2(nu_e) -> Mux2/3
  Selector/1 -> Subsystem2/3(Omega)
  Selector1/1 -> Subsystem7/3(Omega)
  Selector2/1 -> Subsystem8/3(Omega)

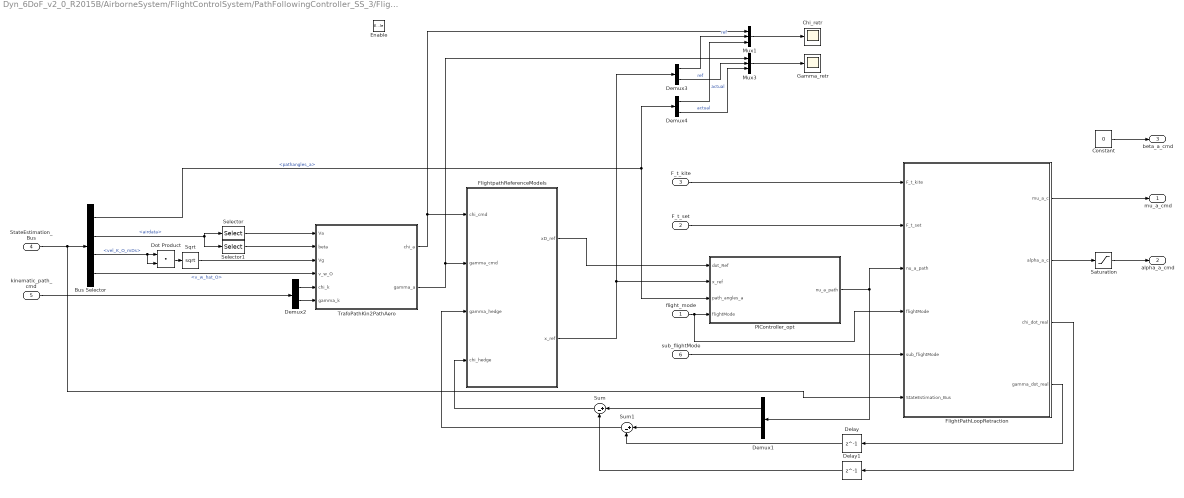
== system Dyn_6DoF_v2_0_R2015B/AirborneSystem/FlightControlSystem/PathFollowingController_SS_3/FlightOnFlatEarth (Retraction&Loitering)/CalculateAttitudeCmds/FlightPathLoopRetraction_Aerodynamic ==
  flight_mode : Inport
  F_t_set : Inport  Port=2
  F_t_kite : Inport  Port=3
  StateEstimation_Bus : Inport  Port=4
  kinematic_path_cmd : Inport  Port=5
  sub_flightMode : Inport  Port=6
  Enable : EnablePort  StatesWhenEnabling=reset
  Bus Selector : BusSelector  OutputSignals=pathangles_a,airdata,vel_K_O_mDs,v_w_hat_O
  Chi_retr : Scope
  Constant : Constant  Value=0
  Delay : Delay  DelayLength=1
  Delay1 : Delay  DelayLength=1
  Demux{1..4} (4 alike) : Demux  Outputs=2
  Dot Product : DotProduct  InputSameDT=on  OutDataTypeStr=Inherit: Inherit via internal rule
  FlightPathLoopRetraction : Subsystem
  FlightpathReferenceModels : Subsystem
  Gamma_retr : Scope
  Mux1 : Mux  Inputs=3
  Mux3 : Mux  Inputs=3
  PIController_opt : Subsystem
  Saturation : Saturate  UpperLimit=constr.alpha_a_max  LowerLimit=constr.alpha_a_min
  Selector : Selector  InputPortWidth=3  IndexOptions=Index vector (dialog)  Indices=1  OutputSizes=1
  Selector1 : Selector  InputPortWidth=3  IndexOptions=Index vector (dialog)  Indices=3  OutputSizes=1
  Sqrt : Sqrt  SaturateOnIntegerOverflow=on
  Sum : Sum  Inputs=|+-
  Sum1 : Sum  Inputs=|+-
  TrafoPathKin2PathAero : MATLAB Function  TreatAsAtomicUnit=on
  mu_a_cmd : Outport
  alpha_a_cmd : Outport  Port=2
  beta_a_cmd : Outport  Port=3
  wires:
  StateEstimation_Bus/1 -> Bus Selector/1, FlightPathLoopRetraction/6(StateEstimation_Bus)
  Bus Selector/1 -> Demux4/1, PIController_opt/3(path_angles_a)  "<pathangles_a>"
  Bus Selector/3 -> Dot Product/2, Dot Product/1  "<vel_K_O_mDs>"
  Bus Selector/2 -> Selector1/1, Selector/1  "<airdata>"
  F_t_kite/1 -> FlightPathLoopRetraction/1(F_t_kite)
  Mux3/1 -> Gamma_retr/1
  Mux1/1 -> Chi_retr/1
  Demux4/1 -> Mux1/3  "actual"
  Demux3/2 -> Mux3/2  "ref"
  Demux4/2 -> Mux3/3  "actual"
  Demux3/1 -> Mux1/2  "ref"
  Demux2/2 -> TrafoPathKin2PathAero/6(gamma_k)
  FlightpathReferenceModels/2(x_ref) -> Demux3/1, PIController_opt/2(x_ref)
  Demux2/1 -> TrafoPathKin2PathAero/5(chi_k)
  FlightPathLoopRetraction/1(mu_a_c) -> mu_a_cmd/1
  FlightpathReferenceModels/1(xD_ref) -> PIController_opt/1(dot_Ref)
  Constant/1 -> beta_a_cmd/1
  FlightPathLoopRetraction/3(chi_dot_real) -> Delay1/1
  PIController_opt/1(nu_a_path) -> FlightPathLoopRetraction/3(nu_a_path), Demux1/1
  Saturation/1 -> alpha_a_cmd/1
  FlightPathLoopRetraction/2(alpha_a_c) -> Saturation/1
  Dot Product/1 -> Sqrt/1
  Sqrt/1 -> TrafoPathKin2PathAero/3(Vg)
  Selector/1 -> TrafoPathKin2PathAero/1(Va)
  TrafoPathKin2PathAero/1(chi_a) -> Mux1/1, FlightpathReferenceModels/1(chi_cmd)
  TrafoPathKin2PathAero/2(gamma_a) -> Mux3/1, FlightpathReferenceModels/2(gamma_cmd)
  Selector1/1 -> TrafoPathKin2PathAero/2(beta)
  F_t_set/1 -> FlightPathLoopRetraction/2(F_t_set)
  kinematic_path_cmd/1 -> Demux2/1
  Bus Selector/4 -> TrafoPathKin2PathAero/4(v_w_O)  "<v_w_hat_O>"
  flight_mode/1 -> PIController_opt/4(flightMode), FlightPathLoopRetraction/4(flightMode)
  FlightPathLoopRetraction/4(gamma_dot_real) -> Delay/1
  Demux1/1 -> Sum/1
  Demux1/2 -> Sum1/1
  Sum/1 -> FlightpathReferenceModels/4(chi_hedge)
  Sum1/1 -> FlightpathReferenceModels/3(gamma_hedge)
  Delay/1 -> Sum1/2
  Delay1/1 -> Sum/2
  sub_flightMode/1 -> FlightPathLoopRetraction/5(sub_flightMode)

== system Dyn_6DoF_v2_0_R2015B/AirborneSystem/FlightControlSystem/PathFollowingController_SS_3/FlightOnFlatEarth (Retraction&Loitering)/GuidanceFlatEarth/LoiteringGuidance ==
  flightMode : Inport
  pos_G_O_m : Inport  Port=2
  vel_K_O_mDs : Inport  Port=3
  pathangles_k : Inport  Port=4
  pos_W : Inport  Port=5
  reset_flag : Inport  Port=6
  Compare To Constant3 : simulink/Logic and Bit Operations/Compare To Constant  relop===  const=1  OutDataTypeStr=boolean
  Constant1 : Constant  Value=ENVMT.windDirection_rad
  Constant3 : Constant  Value=0
  Delay : Delay  DelayLength=1  InitialConditionSource=Input port  ExternalReset=Rising
      settings: InputPortMap=u0,r5,p4
  Delay1 : Delay  DelayLength=1  InitialConditionSource=Input port  ExternalReset=Rising
      settings: InputPortMap=u0,r5,p4
  Dot Product : DotProduct  InputSameDT=on  OutDataTypeStr=Inherit: Inherit via internal rule
  Gain1 : Gain  Gain=-1
  Loiter : Stateflow chart  TreatAsAtomicUnit=on  mask{kp_course_init=loiterStates.kp_delta_course, pos_OLoiter_W=loiterStates.pos_OLoiter_W, R_init_loiter=loiterStates.R, validTransReg_start=loiterStates.validTransReg_start, validTransReg_end=loiterStates.validTransReg_end}
  Mux : Mux  Inputs=2
  Selector1 : Selector  InputPortWidth=2  IndexOptions=Index vector (dialog)  Indices=1  OutputSizes=1
  Selector2 : Selector  InputPortWidth=3  IndexOptions=Index vector (dialog)  Indices=2  OutputSizes=1
  Selector3 : Selector  InputPortWidth=3  IndexOptions=Index vector (dialog)  Indices=1  OutputSizes=1
  Selector4 : Selector  InputPortWidth=3  IndexOptions=Index vector (dialog)  Indices=3  OutputSizes=1
  Sqrt : Sqrt  SaturateOnIntegerOverflow=on
  Subsystem : Subsystem
  Terminator1 : Terminator
  path_k_cmds : Outport
  valid_transition_region : Outport  Port=2
  wires:
  pathangles_k/1 -> Selector1/1
  Mux/1 -> path_k_cmds/1
  Selector1/1 -> Delay/3
  Selector4/1 -> Gain1/1
  Compare To Constant3/1 -> Delay1/2
  pos_W/1 -> Selector2/1, Selector3/1
  Dot Product/1 -> Sqrt/1
  Sqrt/1 -> Loiter/4(Vk)
  Delay1/1 -> Delay1/1, Subsystem/2(h_cmd)
  Loiter/1(course_des) -> Mux/1
  vel_K_O_mDs/1 -> Subsystem/1(v_k_O), Dot Product/1, Dot Product/2
  pos_G_O_m/1 -> Subsystem/3(h), Selector4/1
  Selector3/1 -> Loiter/3(p_x_W)
  Gain1/1 -> Delay1/3
  Subsystem/1(gamma_k_cmd) -> Mux/2
  Delay/1 -> Loiter/2(course_k), Delay/1
  Selector2/1 -> Loiter/1(p_y_W)
  Loiter/2(valid_transition_region_flag) -> valid_transition_region/1
  reset_flag/1 -> Loiter/5(reset_flag)
  Constant1/1 -> Loiter/6(windDir)
  Constant3/1 -> Delay/2
  flightMode/1 -> Compare To Constant3/1
  Loiter/3(e_track) -> Terminator1/1

== system Dyn_6DoF_v2_0_R2015B/AirborneSystem/FlightControlSystem/PathFollowingController_SS_3/FlightOnFlatEarth (Retraction&Loitering)/GuidanceFlatEarth/Retraction_Nav ==
  pos_O : Inport
  vel_k_O : Inport  Port=2
  V_ro : Inport  Port=3
  Tether_length : Inport  Port=4
  Enable : EnablePort  StatesWhenEnabling=reset
  Constant4 : Constant  Value=zeros(3,params.arcPoints)
  Delay : Delay  DelayLength=1
  Delay3 : Delay  DelayLength=1  InitialCondition=zeros(3,params.arcPoints)
  Gain1 : Gain  Gain=pi/180
  Gain2 : Gain  Gain=180/pi
  MATLAB Function1 : MATLAB Function  TreatAsAtomicUnit=on
  Mux : Mux  Inputs=2
  Mux2 : Mux  Inputs=2
  Reshape : Reshape  OutputDimensionality=Row vector (2-D)
  Saturation : Saturate  UpperLimit=constr.gamma_max_retraction  LowerLimit=constr.gamma_min_retraction
  Saturation1 : Saturate  UpperLimit=300  LowerLimit=0
  Scope : Scope  Commented=on  NumInputPorts=2
  Scope1 : Scope  Commented=on
  Subsystem : Subsystem
      mask Display: disp('norm()')
  Vk desired retraction : Scope  Commented=on
  circle_vertical : MATLAB Function  TreatAsAtomicUnit=on
  hold1 : Subsystem
      mask Display: disp('hold()', 'texmode','on')
  distances2slope : Outport
  transition_flag : Outport  Port=2
  flag_pos_y_W : Outport  Port=3
  transition_x_target : Outport  Port=4
  Vk_desired_retraction : Outport  Port=5
  arcP : Outport  Port=6
  path_k_cmds : Outport  Port=7  PortDimensions=[2,1]
  wires:
  circle_vertical/7(gamma_k_cmd) -> Gain2/1
  circle_vertical/8(transition_flag) -> Delay/1, transition_flag/1
  MATLAB Function1/1(vel_k_h_W) -> circle_vertical/7(vk_xy)
  circle_vertical/2(d_gt) -> Mux2/1
  Mux2/1 -> Reshape/1
  circle_vertical/4(chi_k_cmd) -> Mux/1, Scope1/1
  Gain1/1 -> Mux/2
  hold1/1(Out1) -> circle_vertical/5(pos_init_retraction_O)
  circle_vertical/3(d) -> Mux2/2
  vel_k_O/1 -> Subsystem/1(In1), MATLAB Function1/1(vel_k_O)
  Saturation/1 -> Gain1/1, Scope/1
  Mux/1 -> path_k_cmds/1
  Delay/1 -> circle_vertical/9(transition_flag_old)
  Reshape/1 -> distances2slope/1
  circle_vertical/5(flag_pos_y_W) -> flag_pos_y_W/1
  circle_vertical/6(switch_WP_x_W) -> transition_x_target/1
  Gain2/1 -> Saturation/1, Scope/2
  Tether_length/1 -> circle_vertical/4(l_actual)
  V_ro/1 -> circle_vertical/3(V_ro)
  circle_vertical/1(Vk_desired) -> Saturation1/1
  Saturation1/1 -> Vk desired retraction/1, Vk_desired_retraction/1
  Constant4/1 -> circle_vertical/2(arcsize)
  circle_vertical/9(arcP) -> Delay3/1
  Delay3/1 -> circle_vertical/8(arcP_old), arcP/1
  pos_O/1 -> circle_vertical/1(pos_O), hold1/1(In1)
  Subsystem/1(Out1) -> circle_vertical/6(v_k_tot)

== system Dyn_6DoF_v2_0_R2015B/AirborneSystem/FlightControlSystem/PathFollowingController_SS_3/FlightOnSphere (Traction)/FlightPathLoopTraction/EstimatePlantResponse ==
  dphi : Inport
  alpha_rq : Inport  Port=2
  mu_k_sat : Inport  Port=3
  Ft : Inport  Port=4
  StateEstimation_Bus : Inport  Port=5
  Bus Selector : BusSelector  OutputSignals=pathangles_k,pos_G_O_m,v_k_B,airdata
  Demux : Demux  Outputs=2
  MATLAB Function : MATLAB Function  TreatAsAtomicUnit=on
  Mux : Mux  Inputs=3
  Mux4 : Mux  Inputs=2
  Selector : Selector  InputPortWidth=3  IndexOptions=Index vector (dialog)  Indices=1  OutputSizes=1
  Selector1 : Selector  InputPortWidth=3  IndexOptions=Index vector (dialog)  Indices=3  OutputSizes=1
  pathAngleRate : Outport
  wires:
  MATLAB Function/2(gamma_dot_real) -> Mux4/2
  Mux4/1 -> pathAngleRate/1
  MATLAB Function/1(chi_dot_real) -> Mux4/1
  dphi/1 -> MATLAB Function/2(dphi)
  Demux/1 -> MATLAB Function/4(chi_k)
  Demux/2 -> MATLAB Function/5(gamma_k)
  Ft/1 -> MATLAB Function/1(F_t)
  mu_k_sat/1 -> MATLAB Function/3(mu_k)
  StateEstimation_Bus/1 -> Bus Selector/1
  Bus Selector/2 -> MATLAB Function/6(pos_O)  "<pos_G_O_m>"
  Bus Selector/4 -> Selector1/1, Selector/1  "<airdata>"
  Bus Selector/3 -> MATLAB Function/7(v_k_B)  "<v_k_B>"
  Bus Selector/1 -> Demux/1  "<pathangles_k>"
  Selector/1 -> Mux/1
  Selector1/1 -> Mux/3
  alpha_rq/1 -> Mux/2
  Mux/1 -> MATLAB Function/8(airdata)

== system Dyn_6DoF_v2_0_R2015B/AirborneSystem/ForcesAndTorques/aerodynamic forces FSI/Wing Aero/If Action Subsystem1/FSI ==
  In1 : Inport
  1-D Lookup Table : Lookup_n-D  NumberOfTableDimensions=1  BreakpointsForDimension1=DE2019.initAircraft.alpha  BreakpointsForDimension2=[1 1]  Table=DE2019.initAircraft.wing_cL_Static'  InternalRulePriority=Speed  RndMeth=Simplest  InputSameDT=on
  1-D Lookup Table1 : Lookup_n-D  NumberOfTableDimensions=1  BreakpointsForDimension1=DE2019.initAircraft.alpha  BreakpointsForDimension2=[1 1]  Table=DE2019.initAircraft.wing_cD_Static'  InternalRulePriority=Speed  RndMeth=Simplest  InputSameDT=on
  1-D Lookup Table4 : Lookup_n-D  NumberOfTableDimensions=1  BreakpointsForDimension1=DE2019.initAircraft.alpha  BreakpointsForDimension2=[1 1]  Table=DE2019.initAircraft.wing_cM_Static'  InternalRulePriority=Speed  RndMeth=Simplest  InputSameDT=on
  Demux : Demux  Outputs=5
  Gain1 : Gain  Gain=DE2019.initAircraft.wing_cRoll_Static
  Mux6 : Mux  Inputs=6
  Radians to Degrees : simulink_extras/Transformations/Radians to Degrees
  Saturation : Saturate  UpperLimit=max(DE2019.initAircraft.alpha)  LowerLimit=min(DE2019.initAircraft.alpha)
  Saturation3 : Saturate  UpperLimit=act.aileron.max_deflection  LowerLimit=act.aileron.min_deflection
  Simple_wing_aero : MATLAB Function  TreatAsAtomicUnit=on
  Subsystem1 : Subsystem
  Sum3 : Sum  Inputs=+-
  Out1 : Outport
  wires:
  Simple_wing_aero/1(out) -> Out1/1
  In1/1 -> Demux/1
  Mux6/1 -> Simple_wing_aero/1(input)
  Saturation/1 -> 1-D Lookup Table4/1, 1-D Lookup Table1/1, 1-D Lookup Table/1
  Demux/2 -> Subsystem1/1(alpha), Radians to Degrees/1, Mux6/2
  1-D Lookup Table1/1 -> Mux6/4
  1-D Lookup Table/1 -> Mux6/3
  1-D Lookup Table4/1 -> Mux6/5
  Demux/3 -> Subsystem1/2(beta)
  Radians to Degrees/1 -> Saturation/1
  Demux/1 -> Subsystem1/3(velocity), Mux6/1
  Demux/4 -> Subsystem1/4(Omega)
  Demux/5 -> Sum3/1
  Subsystem1/1(defl_damp) -> Sum3/2
  Gain1/1 -> Mux6/6
  Sum3/1 -> Saturation3/1
  Saturation3/1 -> Gain1/1

== system Dyn_6DoF_v2_0_R2015B/AirborneSystem/FlightControlSystem/AttitudeAndRateLoop/RateLoop/Rate_Loop/NonlinearDynamicInversion/Subsystem2 ==
  y_cmd : Inport
  hedge : Inport  Port=2
  Omega : Inport  Port=3
  Roll_PI1 : Subsystem  mask{Kp=Kp, Ki=Ki}
      mask prompts: Kp "Kp_traction"; Ki "Ki_traction"
  SecondOrderReferenceModel_p : Subsystem  mask{omega0_max=w0_max, zeta0=1, y_max=constr.max_rates_B, y_min=-constr.max_rates_B, yd_max=inf, yd_min=-inf, y2d_max=inf, y2d_min=-inf}
  Sum : Sum
  y_ref : Outport
  nu_e : Outport  Port=2
  wires:
  Roll_PI1/1(nu_e) -> Sum/2
  SecondOrderReferenceModel_p/2(y_ref_dot) -> Sum/1
  y_cmd/1 -> SecondOrderReferenceModel_p/1(y_cmd)
  SecondOrderReferenceModel_p/1(y_ref) -> y_ref/1, Roll_PI1/1(p_ref)
  hedge/1 -> SecondOrderReferenceModel_p/2(hedge)
  Sum/1 -> nu_e/1
  Omega/1 -> Roll_PI1/2(p)

== system Dyn_6DoF_v2_0_R2015B/AirborneSystem/FlightControlSystem/AttitudeAndRateLoop/RateLoop/Rate_Loop/NonlinearDynamicInversion/Subsystem7 ==
  y_cmd : Inport
  hedge : Inport  Port=2
  Omega : Inport  Port=3
  Roll_PI1 : Subsystem  mask{Kp=Kp, Ki=Ki}
      mask prompts: Kp "Kp_traction"; Ki "Ki_traction"
  SecondOrderReferenceModel_p : Subsystem  mask{omega0_max=w0_max, zeta0=1, y_max=constr.max_rates_B, y_min=-constr.max_rates_B, yd_max=inf, yd_min=-inf, y2d_max=inf, y2d_min=-inf}
  Sum : Sum
  y_ref : Outport
  nu_e : Outport  Port=2
  wires:
  Roll_PI1/1(nu_e) -> Sum/2
  SecondOrderReferenceModel_p/2(y_ref_dot) -> Sum/1
  y_cmd/1 -> SecondOrderReferenceModel_p/1(y_cmd)
  SecondOrderReferenceModel_p/1(y_ref) -> y_ref/1, Roll_PI1/1(p_ref)
  hedge/1 -> SecondOrderReferenceModel_p/2(hedge)
  Sum/1 -> nu_e/1
  Omega/1 -> Roll_PI1/2(p)

== system Dyn_6DoF_v2_0_R2015B/AirborneSystem/FlightControlSystem/AttitudeAndRateLoop/RateLoop/Rate_Loop/NonlinearDynamicInversion/Subsystem8 ==
  y_cmd : Inport
  hedge : Inport  Port=2
  Omega : Inport  Port=3
  Roll_PI1 : Subsystem  mask{Kp=Kp, Ki=Ki}
      mask prompts: Kp "Kp_traction"; Ki "Ki_traction"
  SecondOrderReferenceModel_p : Subsystem  mask{omega0_max=w0_max, zeta0=1, y_max=constr.max_rates_B, y_min=-constr.max_rates_B, yd_max=inf, yd_min=-inf, y2d_max=inf, y2d_min=-inf}
  Sum : Sum
  y_ref : Outport
  nu_e : Outport  Port=2
  wires:
  Roll_PI1/1(nu_e) -> Sum/2
  SecondOrderReferenceModel_p/2(y_ref_dot) -> Sum/1
  y_cmd/1 -> SecondOrderReferenceModel_p/1(y_cmd)
  SecondOrderReferenceModel_p/1(y_ref) -> y_ref/1, Roll_PI1/1(p_ref)
  hedge/1 -> SecondOrderReferenceModel_p/2(hedge)
  Sum/1 -> nu_e/1
  Omega/1 -> Roll_PI1/2(p)

== system Dyn_6DoF_v2_0_R2015B/AirborneSystem/FlightControlSystem/PathFollowingController_SS_3/FlightOnFlatEarth (Retraction&Loitering)/CalculateAttitudeCmds/FlightPathLoopRetraction_Aerodynamic/FlightPathLoopRetraction ==
  F_t_kite : Inport
  F_t_set : Inport  Port=2
  nu_a_path : Inport  Port=3
  flightMode : Inport  Port=4
  sub_flightMode : Inport  Port=5
  StateEstimation_Bus : Inport  Port=6
  Bus Selector : BusSelector  OutputSignals=pos_G_O_m,pathangles_a,airdata,mu_a
  Chart : Stateflow chart  TreatAsAtomicUnit=on
  Compare To Constant1 : simulink/Logic and Bit Operations/Compare To Constant  relop===  const=7  OutDataTypeStr=boolean
  Compare To Constant2 : simulink/Logic and Bit Operations/Compare To Constant  relop===  const=6  OutDataTypeStr=boolean
  Delay : Delay  DelayLength=1  InitialConditionSource=Input port
      settings: InputPortMap=u0,p4
  Delay1 : Delay  DelayLength=1  InitialConditionSource=Input port
      settings: InputPortMap=u0,p4
  Demux : Demux  Outputs=2
  Demux1 : Demux  Outputs=2
  Logical Operator : Logic  Operator=OR  AllPortsSameDT=off  OutDataTypeStr=boolean
  MATLAB Function : MATLAB Function  TreatAsAtomicUnit=on
  Scope : Scope  NumInputPorts=3
  Scope1 : Scope
  Switch : Switch  Criteria=u2 > Threshold
  Transfer Fcn : TransferFcn  Commented=through  Numerator=[10]  Denominator=[1 10]
  inversionPathDynamics : MATLAB Function  TreatAsAtomicUnit=on
  mu_a_c : Outport  PortDimensions=1
  alpha_a_c : Outport  Port=2  PortDimensions=1
  chi_dot_real : Outport  Port=3  PortDimensions=1
  gamma_dot_real : Outport  Port=4  PortDimensions=1
  wires:
  Bus Selector/1 -> inversionPathDynamics/6(pos_O)  "<pos_G_O_m>"
  Demux1/2 -> inversionPathDynamics/8(gamma_a)
  Bus Selector/2 -> Demux1/1  "<pathangles_a>"
  Bus Selector/3 -> inversionPathDynamics/9(airdata), MATLAB Function/1(airdata)  "<airdata>"
  StateEstimation_Bus/1 -> Bus Selector/1
  MATLAB Function/1(L_rq) -> Delay/2
  inversionPathDynamics/1(mu_a_c) -> Delay1/1, mu_a_c/1
  Delay1/1 -> inversionPathDynamics/1(mu_a_c_old)
  Delay/1 -> inversionPathDynamics/11(Lrq_old)
  flightMode/1 -> inversionPathDynamics/3(flightMode)
  nu_a_path/1 -> Demux/1
  Demux/2 -> inversionPathDynamics/5(nu_gamma_a)
  Demux/1 -> inversionPathDynamics/4(nu_chi_a)
  inversionPathDynamics/2(alpha_a_c) -> alpha_a_c/1
  Demux1/1 -> inversionPathDynamics/7(chi_a)
  Bus Selector/4 -> inversionPathDynamics/10(mu_a), Delay1/2  "<mu_a>"
  inversionPathDynamics/5(L_rq) -> Delay/1
  inversionPathDynamics/3(chi_dot_real) -> chi_dot_real/1
  inversionPathDynamics/4(gamma_dot_real) -> gamma_dot_real/1
  F_t_set/1 -> Scope/1, Chart/1(Ftset)
  F_t_kite/1 -> Switch/1, Chart/2(Ftm)
  Chart/1(fset) -> Switch/3, Scope/2
  Switch/1 -> Scope/3, inversionPathDynamics/2(f_t)
  sub_flightMode/1 -> Scope1/1, Chart/3(sub_flightMode), Compare To Constant1/1, Compare To Constant2/1
  Compare To Constant2/1 -> Logical Operator/2
  Compare To Constant1/1 -> Logical Operator/1
  Logical Operator/1 -> Switch/2

== system Dyn_6DoF_v2_0_R2015B/AirborneSystem/FlightControlSystem/PathFollowingController_SS_3/FlightOnFlatEarth (Retraction&Loitering)/CalculateAttitudeCmds/FlightPathLoopRetraction_Aerodynamic/FlightpathReferenceModels ==
  chi_cmd : Inport
  gamma_cmd : Inport  Port=2
  gamma_hedge : Inport  Port=3
  chi_hedge : Inport  Port=4
  Mux2 : Mux  Inputs=2
  Mux3 : Mux  Inputs=2
  SecondOrderReferenceModel_course : Subsystem  mask{omega0_max=params.w0_chi_retraction_max, zeta0=1, y_max=inf, y_min=-inf, yd_max=inf, yd_min=-inf, y2d_max=inf, y2d_min=-inf}
  SecondOrderReferenceModel_pathangle : Subsystem  mask{omega0_max=params.w0_gamma_retraction_max, zeta0=1, y_max=inf, y_min=-inf, yd_max=inf, yd_min=-inf, y2d_max=inf, y2d_min=-inf}
  xD_ref : Outport
  x_ref : Outport  Port=2
  wires:
  gamma_hedge/1 -> SecondOrderReferenceModel_pathangle/2(hedge)
  chi_hedge/1 -> SecondOrderReferenceModel_course/2(hedge)
  gamma_cmd/1 -> SecondOrderReferenceModel_pathangle/1(y_cmd)
  chi_cmd/1 -> SecondOrderReferenceModel_course/1(y_cmd)
  Mux3/1 -> xD_ref/1
  Mux2/1 -> x_ref/1
  SecondOrderReferenceModel_course/1(y_ref) -> Mux2/1
  SecondOrderReferenceModel_pathangle/1(y_ref) -> Mux2/2
  SecondOrderReferenceModel_course/2(y_ref_dot) -> Mux3/1
  SecondOrderReferenceModel_pathangle/2(y_ref_dot) -> Mux3/2
